simulink subsystem "rss_DycAmpCmpt"  (R2023a)
settings: Solver=VariableStepAuto  StartTime=0.0  StopTime=10.0  RelTol=1e-3
undefined symbols (not defined in the file): Cdbl_uPhVltgMaxVal
libraries: simulink x1, lib_conversion x1
settings Model: DefaultTestHarness=rss_DutyCycleAmplitudeComputation_thu  Creator=CAV2OFO  LastModifiedBy=xiaoqiang.yuan
settings OptimizationCC: ReuseModelBlockBuffer=off

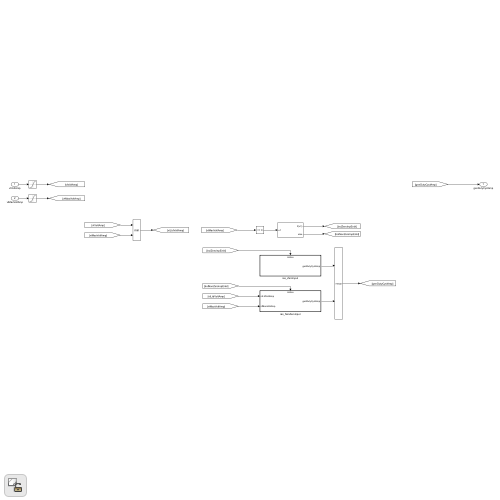
[thumbnail: Simulink's stored preview of the top-level diagram]
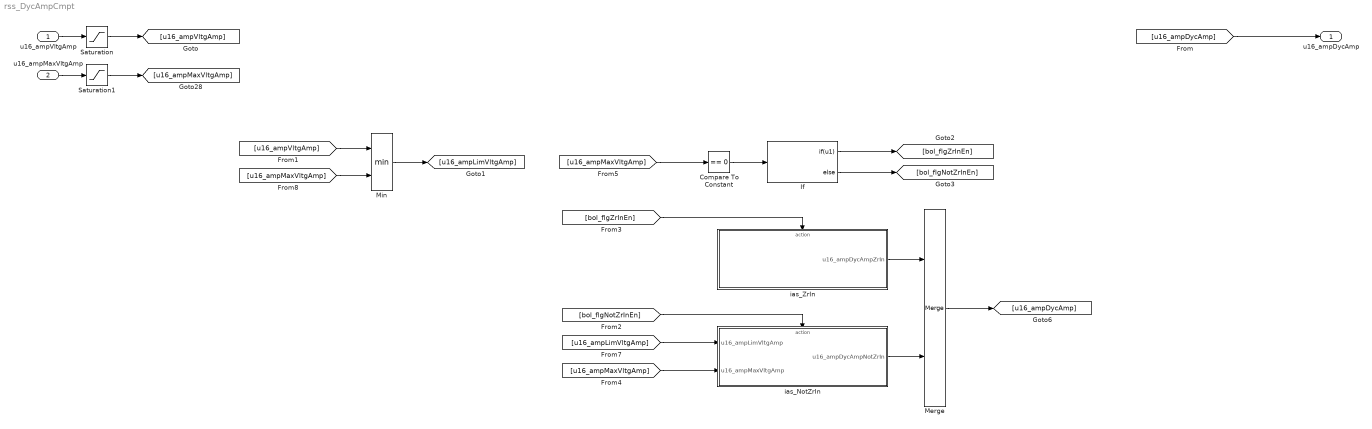
== system rss_DycAmpCmpt ==
  u16_ampVltgAmp : Inport  OutDataTypeStr=dt_Standardize_u16p15b0
  u16_ampMaxVltgAmp : Inport  Port=2  OutDataTypeStr=dt_Standardize_u16p15b0
  Compare To Constant : simulink/Logic and Bit Operations/Compare To Constant  relop===  const=0  OutDataTypeStr=boolean
  If : If  IfExpression=u1
  Merge : Merge
  Min : MinMax  Inputs=2  RndMeth=Simplest
  Saturation : Saturate  UpperLimit=Cdbl_uPhVltgMaxVal  LowerLimit=0
  Saturation1 : Saturate  UpperLimit=Cdbl_uPhVltgMaxVal  LowerLimit=0
  ias_NotZrIn : Subsystem  TreatAsAtomicUnit=on
  ias_ZrIn : Subsystem  TreatAsAtomicUnit=on
  u16_ampDycAmp : Outport  OutDataTypeStr=dt_DutyCycl_u16p15b0
  wires:
  Min/1 -> [u16_ampLimVltgAmp]
  [u16_ampMaxVltgAmp] -> Min/2
  [u16_ampVltgAmp] -> Min/1
  u16_ampMaxVltgAmp/1 -> Saturation1/1
  [bol_flgNotZrInEn] -> ias_NotZrIn/Action
  If/2 -> [bol_flgNotZrInEn]
  [bol_flgZrInEn] -> ias_ZrIn/Action
  If/1 -> [bol_flgZrInEn]
  [u16_ampDycAmp] -> u16_ampDycAmp/1
  Merge/1 -> [u16_ampDycAmp]
  ias_NotZrIn/1(u16_ampDycAmpNotZrIn) -> Merge/2
  ias_ZrIn/1(u16_ampDycAmpZrIn) -> Merge/1
  [u16_ampLimVltgAmp] -> ias_NotZrIn/1(u16_ampLimVltgAmp)
  u16_ampVltgAmp/1 -> Saturation/1
  [u16_ampMaxVltgAmp] -> ias_NotZrIn/2(u16_ampMaxVltgAmp)
  Compare To Constant/1 -> If/1
  [u16_ampMaxVltgAmp] -> Compare To Constant/1
  Saturation/1 -> [u16_ampVltgAmp]
  Saturation1/1 -> [u16_ampMaxVltgAmp]

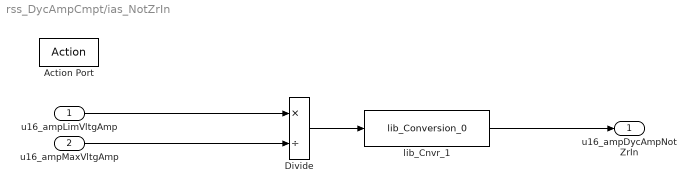
== system rss_DycAmpCmpt/ias_NotZrIn ==
  u16_ampLimVltgAmp : Inport
  u16_ampMaxVltgAmp : Inport  Port=2
  Action Port : ActionPort
  Divide : Product  Inputs=*/  OutDataTypeStr=Inherit: Inherit via back propagation  RndMeth=Simplest
  lib_Cnvr_1 : lib_conversion/lib_Conversion_0  lb_parDataType=dt_DutyCycl_u16p15b0  lb_parOutpMaxVal=[]  lb_parOutpMinVal=[]  lb_parSatFlag=off
  u16_ampDycAmpNotZrIn : Outport
  wires:
  u16_ampLimVltgAmp/1 -> Divide/1
  lib_Cnvr_1/1 -> u16_ampDycAmpNotZrIn/1
  Divide/1 -> lib_Cnvr_1/1
  u16_ampMaxVltgAmp/1 -> Divide/2

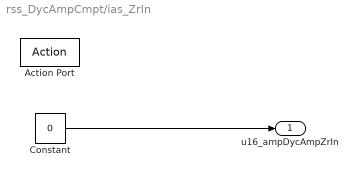
== system rss_DycAmpCmpt/ias_ZrIn ==
  Action Port : ActionPort
  Constant : Constant  Value=0  OutDataTypeStr=dt_DutyCycl_u16p15b0
  u16_ampDycAmpZrIn : Outport
  wires:
  Constant/1 -> u16_ampDycAmpZrIn/1
